simulink model "Outer_Loop_Linear_DCM_Torque_Input"  (R2024b)
settings: Solver=ode15s  StartTime=0.0  StopTime=stop_time  RelTol=1e-5  AbsTol=1e-7
undefined symbols (not defined in the file or in its folder): ctrl, F_wq_s, G_iv_s, G_wv_s, t_step, time_shift, Ts, w_ref_start, w_ref_stop
libraries: cstblocks x6
settings Model: SimulationMode=accelerator  Creator=rs  LastModifiedBy=matth
settings SolverCC: AutoScaleAbsTol=off  ZeroCrossAlgorithm=Adaptive  AlgebraicLoopSolver=TrustRegion
settings DataIOCC: SaveFormat=Array  SaveOutput=off  SignalLogging=off  DSMLogging=off  SaveTime=off  ReturnWorkspaceOutputs=off  TimeSaveName=t  OutputSaveName=y
settings DebuggingCC: UnconnectedInputMsg=warning  UnconnectedOutputMsg=warning  UnconnectedLineMsg=warning  ArithmeticOperatorsInVariantConditions=warning
settings ModelReferenceCC: EnableRefExpFcnMdlSchedulingChecks=on
settings SFSimCC: SimUseLocalCustomCode=off  CustomCodeUndefinedFunction=UseInterfaceOnly
settings RTWCC: RTWUseLocalCustomCode=off  GPUComputeCapability=3.5

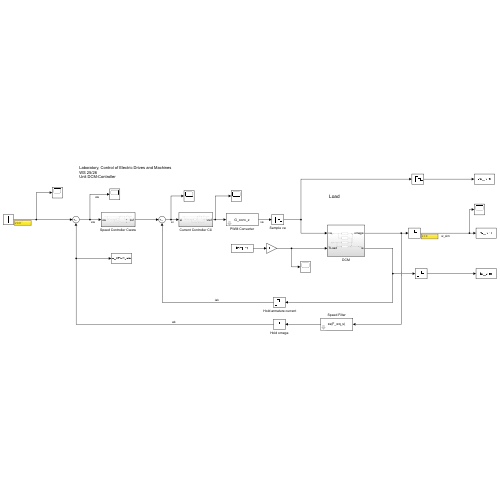
[thumbnail: Simulink's stored preview of the top-level diagram]
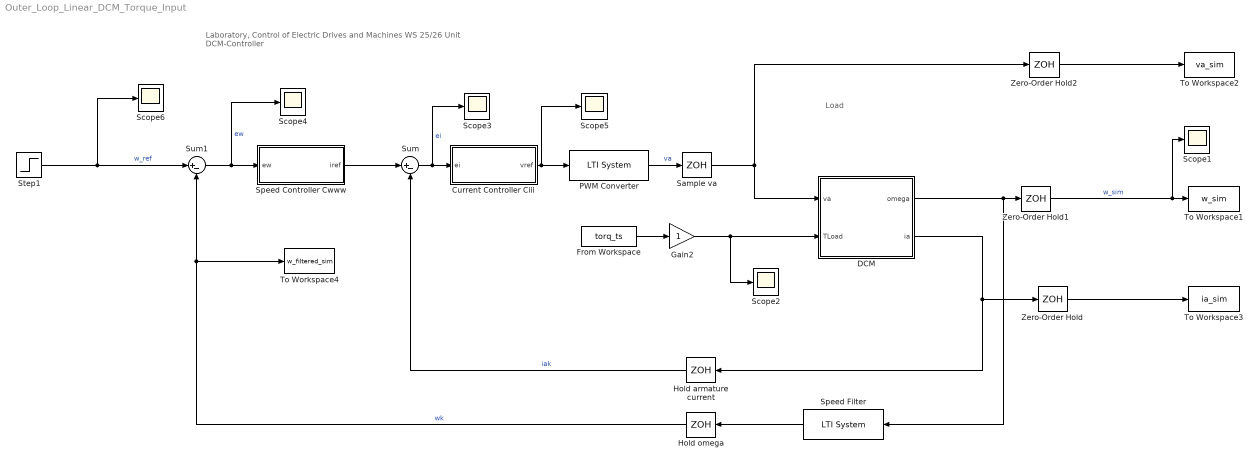
== system Outer_Loop_Linear_DCM_Torque_Input ==
  note: Laboratory, Control of Electric Drives and Machines
      | WS 25/26
      | Unit DCM-Controller
  note: Load
  " Hold armature current" : ZeroOrderHold  SampleTime=-1
  Current Controller Ciii : Subsystem
  DCM : Subsystem
  From Workspace : FromWorkspace  VariableName=torq_ts  SampleTime=Ts
  Gain2 : Gain
  Hold omega : ZeroOrderHold  SampleTime=-1
  PWM Converter : cstblocks/LTI System  sys=G_conv_z  IC=[]  PadeOrder=0
  Sample va : ZeroOrderHold  SampleTime=-1
  Scope{1..6} (6 alike) : Scope
  Speed Controller Cwww : Subsystem
  Speed Filter : cstblocks/LTI System  sys=ss(F_wq_s)  IC=w0  PadeOrder=0
      link override Internal: InitialCondition=w_start
  Step1 : Step  Time=t_step + time_shift  Before=w_ref_start  After=w_ref_stop  SampleTime=0  VectorParams1D=off
  Sum : Sum  Inputs=|+-
  Sum1 : Sum  Inputs=|+-
  To Workspace1 : ToWorkspace  VariableName=w_sim  SaveFormat=Timeseries  SampleTime=-1
  To Workspace2 : ToWorkspace  VariableName=va_sim  SaveFormat=Timeseries  SampleTime=-1
  To Workspace3 : ToWorkspace  VariableName=ia_sim  SaveFormat=Timeseries  SampleTime=-1
  To Workspace4 : ToWorkspace  VariableName=w_filtered_sim  SaveFormat=Timeseries  SampleTime=-1
  Zero-Order Hold : ZeroOrderHold  SampleTime=Ts
  Zero-Order Hold1 : ZeroOrderHold  SampleTime=Ts
  Zero-Order Hold2 : ZeroOrderHold  SampleTime=Ts
  wires:
  Zero-Order Hold/1 -> To Workspace3/1
  Zero-Order Hold2/1 -> To Workspace2/1
  Sum/1 -> Scope3/1, Current Controller Ciii/1(ei)  "ei"
  " Hold armature current"/1 -> Sum/2  "iak"
  Speed Controller Cwww/1(iref) -> Sum/1
  Sample va/1 -> DCM/1(va), Zero-Order Hold2/1
  PWM Converter/1 -> Sample va/1  "va"
  Current Controller Ciii/1(vref) -> Scope5/1, PWM Converter/1
  Sum1/1 -> Scope4/1, Speed Controller Cwww/1(ew)  "ew"
  Hold omega/1 -> To Workspace4/1, Sum1/2  "wk"
  Speed Filter/1 -> Hold omega/1
  Step1/1 -> Scope6/1, Sum1/1  "w_ref"
  DCM/1(omega) -> Zero-Order Hold1/1, Speed Filter/1
  DCM/2(ia) -> " Hold armature current"/1, Zero-Order Hold/1
  From Workspace/1 -> Gain2/1
  Gain2/1 -> DCM/2(TLoad), Scope2/1
  Zero-Order Hold1/1 -> Scope1/1, To Workspace1/1  "w_sim"

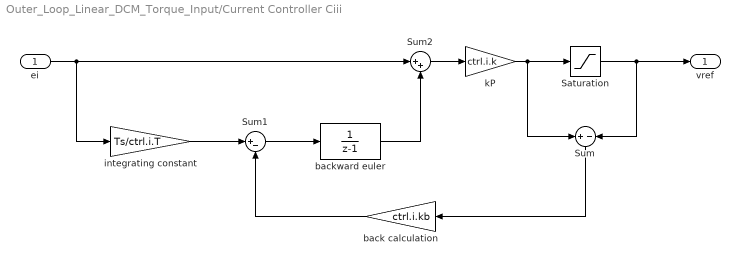
== system Outer_Loop_Linear_DCM_Torque_Input/Current Controller Ciii ==
  ei : Inport
  Saturation : Saturate  UpperLimit=120  LowerLimit=-120
  Sum : Sum  Inputs=+|-
  Sum1 : Sum  Inputs=|+-
  Sum2 : Sum  Inputs=|++
  back calculation : Gain  Gain=ctrl.i.kb
  backward euler : DiscreteTransferFcn  Denominator=[1 -1]
  integrating constant : Gain  Gain=Ts/ctrl.i.T
  kP : Gain  Gain=ctrl.i.k
  vref : Outport
  wires:
  Sum1/1 -> backward euler/1
  integrating constant/1 -> Sum1/1
  Saturation/1 -> vref/1, Sum/2
  Sum/1 -> back calculation/1
  back calculation/1 -> Sum1/2
  ei/1 -> integrating constant/1, Sum2/1
  Sum2/1 -> kP/1
  kP/1 -> Sum/1, Saturation/1
  backward euler/1 -> Sum2/2

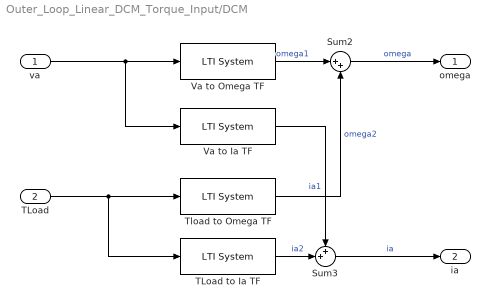
== system Outer_Loop_Linear_DCM_Torque_Input/DCM ==
  va : Inport
  TLoad : Inport  Port=2
  Sum2 : Sum  Inputs=|++
  Sum3 : Sum  Inputs=++|
  TLoad to Ia TF : cstblocks/LTI System  sys=G_iT_s  IC=ia0  PadeOrder=0
  Tload to Omega TF : cstblocks/LTI System  sys=G_wT_s  IC=[]  PadeOrder=0
  Va to Ia TF : cstblocks/LTI System  sys=ss(G_iv_s)  IC=ia0  PadeOrder=0
  Va to Omega TF : cstblocks/LTI System  sys=ss(G_wv_s)  IC=w0  PadeOrder=0
      link override Internal: InitialCondition=w_start
  omega : Outport
  ia : Outport  Port=2
  wires:
  Sum2/1 -> omega/1  "omega"
  TLoad to Ia TF/1 -> Sum3/2  "ia2"
  TLoad/1 -> TLoad to Ia TF/1, Tload to Omega TF/1
  Va to Omega TF/1 -> Sum2/1  "omega1"
  Va to Ia TF/1 -> Sum3/1  "ia1"
  Tload to Omega TF/1 -> Sum2/2  "omega2"
  va/1 -> Va to Ia TF/1, Va to Omega TF/1
  Sum3/1 -> ia/1  "ia"

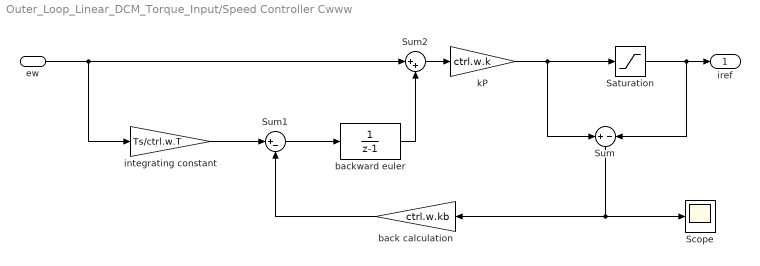
== system Outer_Loop_Linear_DCM_Torque_Input/Speed Controller Cwww ==
  ew : Inport
  Saturation : Saturate  UpperLimit=30  LowerLimit=-30
  Scope : Scope
  Sum : Sum  Inputs=+|-
  Sum1 : Sum  Inputs=|+-
  Sum2 : Sum  Inputs=|++
  back calculation : Gain  Gain=ctrl.w.kb
  backward euler : DiscreteTransferFcn  Denominator=[1 -1]
  integrating constant : Gain  Gain=Ts/ctrl.w.T
  kP : Gain  Gain=ctrl.w.k
  iref : Outport
  wires:
  ew/1 -> Sum2/1, integrating constant/1
  backward euler/1 -> Sum2/2
  Saturation/1 -> iref/1, Sum/2
  back calculation/1 -> Sum1/2
  integrating constant/1 -> Sum1/1
  kP/1 -> Sum/1, Saturation/1
  Sum2/1 -> kP/1
  Sum1/1 -> backward euler/1
  Sum/1 -> back calculation/1, Scope/1
